simulink subsystem "Motors"  (R2024a)
settings: Solver=VariableStepAuto  StartTime=0.0  StopTime=10.0  RelTol=1e-3
libraries: stm32l4xxblockslib x2, stm32f4xxblockslib x1
settings Model: Creator=JesseJabezArendse  LastModifiedBy=user
settings RTWCC: GPUComputeCapability=3.5

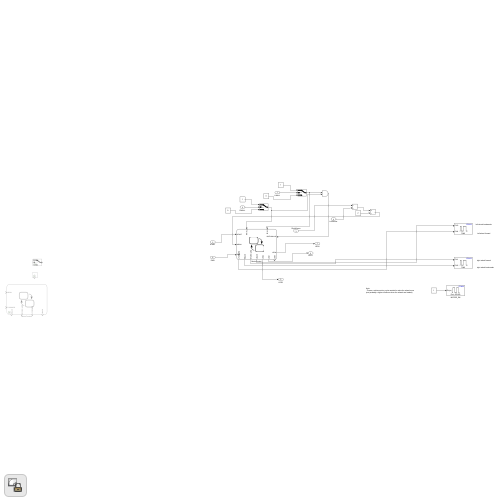
[thumbnail: Simulink's stored preview of the top-level diagram]
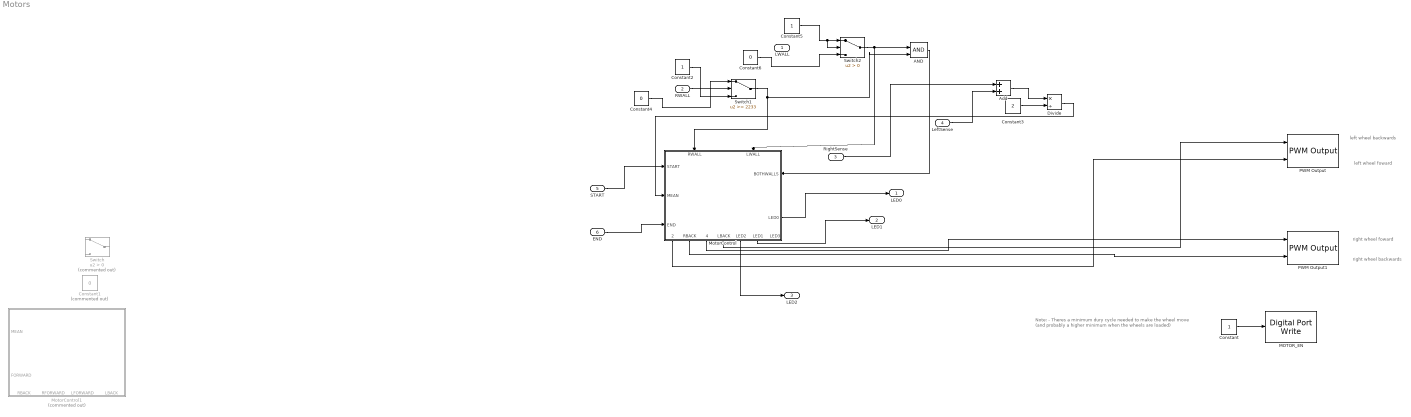
== system Motors ==
  note: Note:
      | - Theres a minimum dury cycle needed to make the wheel move (and probably a higher minimum when the wheels are loaded)
  note: left wheel foward
  note: left wheel backwards
  note: right wheel backwards
  note: right wheel foward
  LWALL : Inport
  RWALL : Inport  Port=2
  RightSense : Inport  Port=3
  LeftSense : Inport  Port=4
  START : Inport  Port=5
  END : Inport  Port=6
  AND : Logic  IconShape=distinctive  AllPortsSameDT=off  OutDataTypeStr=boolean
  Add : Sum
  Constant : Constant
  Constant1 : Constant  Commented=on  Value=0
  Constant2 : Constant
  Constant3 : Constant  Value=2
  Constant4 : Constant  Value=0
  Constant5 : Constant
  Constant6 : Constant  Value=0
  Divide : Product  Inputs=*/
  MOTOR_EN : stm32f4xxblockslib/Digital Port Write  PortName=GPIOD  PinNumber=7  ReadOperation=off  IOAsArray=on  EnableSimPort=off  hoistedMaskSrc=ECSoC/ECSimCodegen/Digital Port Write
      settings: LibrarySourceBlock=stm32l4xxblockslib/Digital Port Write
  MotorControl : Stateflow chart  TreatAsAtomicUnit=on
      settings: PortSchema="{\"entries\":[{\"content\":{\"sides\":[{\"content\":{\"connectorIds\":[\"In5\",\"In6\",\"In4\"]},\"type\":\"ConnectorPlacement.EquallySpacedRectSide\",\"uuid\":\"f52daa4f-6374-42e5-9ef1-0ccc99d09b58\"},{\"content\":{\"connectorIds\":[\"In1\",\"Out1\"],\"side\":\"RIGHT\"},\"type\":\"ConnectorPlacement.EquallySpacedRectSide\",\"uuid\":\"94b478cc-4dde-45c7-a588-77cf2b43cdb7\"},{\"content\":{\"connectorIds\":[\"In2\",\"In3\"],\"side\":\"TOP\"},\"type\":\"ConnectorPlacement.EquallySpacedRectSide\",\"uuid\":\"afff2079-ea5c-423e-9722-09c3bbce433b\"},{\"content\":{\"connectorIds\":[\"Out2\",\"Out3\",\"Out4\",\"Out5\",\"Out6\",\"Out7\",\"Out8\"],\"side\":\"BOTTOM\"},\"type\":\"ConnectorPlacement.EquallySpacedRectSide\",\"uuid\":\"94e93a1d-795d-41a3-b2d8-d520b2bf47ef\"}]},\"type\":\"ConnectorPlacement.EquallySpacedConnector\",\"uuid\":\"d4d35636-54af-48ac-af70-d56caef5e090\"}],\"packageUris\":[\"http://schema.mathworks.com/mf0/Connector/R2020b\"],\"version\":\"1.0\"}"
  MotorControl1 : Stateflow chart  Commented=on  TreatAsAtomicUnit=on
      settings: PortSchema="{\"entries\":[{\"content\":{\"sides\":[{\"content\":{\"connectorIds\":[\"In2\",\"In1\"]},\"type\":\"ConnectorPlacement.EquallySpacedRectSide\",\"uuid\":\"f52daa4f-6374-42e5-9ef1-0ccc99d09b58\"},{\"content\":{\"side\":\"RIGHT\"},\"type\":\"ConnectorPlacement.EquallySpacedRectSide\",\"uuid\":\"94b478cc-4dde-45c7-a588-77cf2b43cdb7\"},{\"content\":{\"side\":\"TOP\"},\"type\":\"ConnectorPlacement.EquallySpacedRectSide\",\"uuid\":\"afff2079-ea5c-423e-9722-09c3bbce433b\"},{\"content\":{\"connectorIds\":[\"Out1\",\"Out2\",\"Out3\",\"Out4\"],\"side\":\"BOTTOM\"},\"type\":\"ConnectorPlacement.EquallySpacedRectSide\",\"uuid\":\"94e93a1d-795d-41a3-b2d8-d520b2bf47ef\"}]},\"type\":\"ConnectorPlacement.EquallySpacedConnector\",\"uuid\":\"d4d35636-54af-48ac-af70-d56caef5e090\"}],\"packageUris\":[\"http://schema.mathworks.com/mf0/Connector/R2020b\"],\"version\":\"1.0\"}"
  PWM Output : stm32l4xxblockslib/PWM Output  TimerModule=TIM3  DutycycleUnits=Counts  EnableChannel1=off  EnableChannel2=off  EnableChannel3=on  EnableChannel4=on  EnableChannel5=off  EnableChannel6=off  EnableCounterInput=off  EnableMainOutputInput=off  EnableFrequencyInput=off  SetRCAfterCE=off  OutputDirection=off  OutputMainOutputEnableStatus=off  SampleTime=0.1  EnableSimPort=off  EnableUpdateEvent=off  EnableCaptureCompare1Event=off  EnableCaptureCompare2Event=off  EnableCaptureCompare3Event=off  EnableCaptureCompare4Event=off  EnableTriggerEvent=off  EnableBreakEvent=off  EnableBreakEvent2=off  ProcessorFamily=STM32L4  hoistedMaskSrc=ECSoC/ECSimCodegen/PWM Output
  PWM Output1 : stm32l4xxblockslib/PWM Output  TimerModule=TIM3  DutycycleUnits=Counts  EnableChannel1=on  EnableChannel2=on  EnableChannel3=off  EnableChannel4=off  EnableChannel5=off  EnableChannel6=off  EnableCounterInput=off  EnableMainOutputInput=off  EnableFrequencyInput=off  SetRCAfterCE=off  OutputDirection=off  OutputMainOutputEnableStatus=off  SampleTime=0.1  EnableSimPort=off  EnableUpdateEvent=off  EnableCaptureCompare1Event=off  EnableCaptureCompare2Event=off  EnableCaptureCompare3Event=off  EnableCaptureCompare4Event=off  EnableTriggerEvent=off  EnableBreakEvent=off  EnableBreakEvent2=off  ProcessorFamily=STM32L4  hoistedMaskSrc=ECSoC/ECSimCodegen/PWM Output
  Switch : Switch  Commented=on  Criteria=u2 > Threshold  SaturateOnIntegerOverflow=off  InputSameDT=off
  Switch1 : Switch  Threshold=2233  SaturateOnIntegerOverflow=off  InputSameDT=off
  Switch2 : Switch  Criteria=u2 > Threshold  SaturateOnIntegerOverflow=off  InputSameDT=off
  LED0 : Outport
  LED1 : Outport  Port=2
  LED2 : Outport  Port=3
  wires:
  Constant/1 -> MOTOR_EN/1
  START/1 -> MotorControl/5(START)
  END/1 -> MotorControl/4(END)
  RightSense/1 -> Add/1
  LeftSense/1 -> Add/2
  Add/1 -> Divide/1
  Constant3/1 -> Divide/2
  Divide/1 -> MotorControl/6(MEAN)
  MotorControl/5(LBACK) -> PWM Output/1
  MotorControl/2(LFORWARD) -> PWM Output/2
  MotorControl/4(RFORWARD) -> PWM Output1/1
  MotorControl/3(RBACK) -> PWM Output1/2
  RWALL/1 -> Switch1/2
  Switch1/1 -> MotorControl/2(RWALL), AND/2
  Constant2/1 -> Switch1/3
  Constant4/1 -> Switch1/1
  Switch2/1 -> AND/1, MotorControl/3(LWALL)
  Constant6/1 -> Switch2/3
  Constant5/1 -> Switch2/1, Switch2/2
  AND/1 -> MotorControl/1(BOTHWALLS)
  MotorControl/6(LED2) -> LED2/1
  MotorControl/7(LED1) -> LED1/1
  MotorControl/1(LED0) -> LED0/1

== stateflow chart Motors/MotorControl ==
  state WaitUntilButtonPressed
    during:
    LED0=0;
    LED1=0;
    LED2=0;
  state STOP
    during:
    RFORWARD=0;
    RBACK=0;
    LFORWARD=0;
    LBACK=0;
    LED0=0;
    LED1=0;
    LED2=0;
  state FORWARDMOVE
    during:
    state STRAIGHT
      during:
      RFORWARD=(2^16 -1)*0.7;
      RBACK=0;
      LFORWARD=(2^16 -1)*0.7;
      LBACK=0;
    state COMPLETE [commented out]
      during:
      LED0=1;
      LED1=1;
      LED2=1;
      RFORWARD=0;
      RBACK=0;
      LFORWARD=0;
      LBACK=0;
    state TURNENTRY
      during:
      LED3=1;
      LED0=0;
      LED1=0;
      LED2=0;
    state CHECKCOMPLETE [commented out]
      during:
      LED3=1;
      CHECKCOMPLETE -> CHECKCOMPLETE [commented out]
    state TURNRIGHT
      during:
      LFORWARD=(2^16 -1)*0.4;
      LBACK=0;
      RFORWARD=0;
      RBACK=(2^16 -1)*0.4;
    state TURNLEFT [commented out]
      during:
      RFORWARD=(2^16 -1)*0.4;
      RBACK=0;
      LFORWARD=0;
      LBACK=(2^16 -1)*0.4;
    STRAIGHT -> TURNRIGHT : [MEAN>=3226]
    (default) -> TURNENTRY
    TURNENTRY -> STRAIGHT [order 2] : [MEAN<3226]
    TURNRIGHT -> TURNENTRY : after(0.3,sec)
    TURNENTRY -> TURNRIGHT [order 1] : [MEAN>=3226]
  (default) -> WaitUntilButtonPressed
  WaitUntilButtonPressed -> FORWARDMOVE : [START]
  FORWARDMOVE -> STOP : [END]
  STOP -> FORWARDMOVE : [START]
  data: BOTHWALLS input; RWALL input; LWALL input; END input; LED0 output; START input; LFORWARD output; RBACK output; RFORWARD output; MEAN input; LBACK output; LED2 output; LED1 output; LED3 output

== stateflow chart Motors/MotorControl1 ==
  state WaitUntilButtonPressed
    during:
    RFORWARD=0;
    RBACK=0;
    LFORWARD=0;
    LBACK=0;
  state FORWARDMOVE
    during:
    if MEAN>=2.2
    RFORWARD=(2^16 -1)*0.7;
    RBACK=0;
    LFORWARD=0;
    LBACK=(2^16 -1)*0.7;
    else
    RFORWARD=(2^16 -1)*0.7;
    RBACK=0;
    LFORWARD=(2^16 -1)*0.7;
    LBACK=0;
    end
  FORWARDMOVE -> WaitUntilButtonPressed : [FORWARD==0]
  WaitUntilButtonPressed -> FORWARDMOVE : [FORWARD]
  (default) -> (junction 32) [order 2]
  (default) -> FORWARDMOVE [order 1] : [FORWARD]
  data: FORWARD input; MEAN input; RBACK output; RFORWARD output; LFORWARD output; LBACK output
